simulink model "control_project2"  (R2015a)
settings: Solver=ode45  StartTime=0.0  StopTime=10.0  RelTol=1e-3
libraries: simulink x2
settings Model: Creator=Farhan Fuad  LastModifiedBy=Farhan Fuad

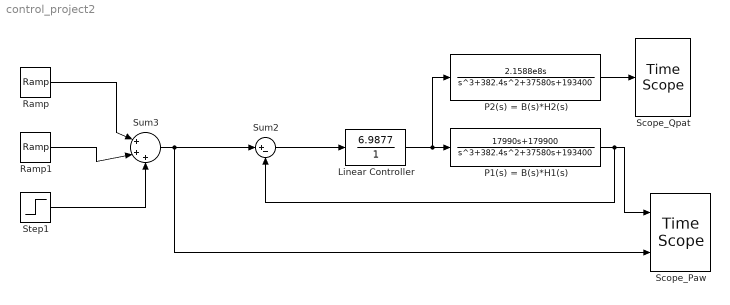
== system control_project2 ==
  Linear Controller : TransferFcn  Numerator=[6.9877]  Denominator=[1 ]
  P1(s) = B(s)*H1(s) : TransferFcn  Numerator=[0 0 17990 179900]  Denominator=[1 382.4 37580 193400]
  P2(s) = B(s)*H2(s) : TransferFcn  Numerator=[0 0 2.1588e8 0]  Denominator=[1 382.4 37580 193400]
  Ramp : simulink/Sources/Ramp  slope=64.865  start=1  X0=0
  Ramp1 : simulink/Sources/Ramp  slope=-64.865  start=1.23125  X0=0
  "Scope_Paw " : TimeScope  NumInputPorts=2
  Scope_Qpat : TimeScope
  Step1 : Step  Time=5  After=-15  SampleTime=0
  Sum2 : Sum  Inputs=|+-
  Sum3 : Sum  Inputs=|+++
  wires:
  Ramp/1 -> Sum3/1
  Ramp1/1 -> Sum3/2
  Sum2/1 -> Linear Controller/1
  Sum3/1 -> "Scope_Paw "/2, Sum2/1
  P2(s) = B(s)*H2(s)/1 -> Scope_Qpat/1
  P1(s) = B(s)*H1(s)/1 -> "Scope_Paw "/1, Sum2/2
  Step1/1 -> Sum3/3
  Linear Controller/1 -> P2(s) = B(s)*H2(s)/1, P1(s) = B(s)*H1(s)/1
